simulink model "AEBMIL"  (Simulink 8.2)
settings: Solver=FixedStepDiscrete  StartTime=0.0  StopTime=126  FixedStep=0.005  RelTol=1e-3
PostLoadFcn:
  | , if any(exist('dsrtsu_mdlpostloadfcn', 'file') == [2, 3, 6]), try dsrtsu_mdlpostloadfcn('Execute', bdroot); catch fprintf('Error in PostLoadFcn (dsrtsu_mdlpostloadfcn) for model "%s":\n %s\n', bdroot, lasterr); end, end,
values from neighbouring files (symbols this model uses):
  C_TASK_5MS_S = (	C_TICK_TIME_S      	)    [hcu_local_hdr.m]
  ENUM_GEARPOSN_1ST = uint8(  1  )    [hcu_local_hdr.m]
  ENUM_GEARPOSN_R = uint8(  7  )    [hcu_local_hdr.m]
  FALSE = boolean( 0 )    [hcu_local_hdr.m]
  R_OBJ_Position = single([ii 0 0])    [GridSearch.m]
  R_OBJ_RelAccel = single([0 0 kk])    [GridSearch.m]
  R_OBJ_RelVelocity = single([0 jj 0])    [GridSearch.m]
  TRUE = boolean( 1 )    [hcu_local_hdr.m]
undefined symbols (not defined in the file or in its folder): A_OBJ, AAEB_VehSpd_kph, B_OBJ, C_OBJ, Gamma_OBJ, KAEB_AEBActiveCount_cnt, KAEB_DsblAEBAPPRateThres_pctps, KAEB_DsblAEBSteerRateThres_degps, KAEB_UseMCTTTC_flg, KAEB_VehHoldSpdThres_kph, KOBJ_KalmanFilterCalRate_s, KOBJ_UseCalObjSpd_flg, KOBJ_UseEstObjInfo_flg, KOBJ_VehAccCalRate_s, KOBJ_VehAccFltConst_s, KPTH_ObjPositionYLimit_m, MAEB_AEBTTCThres_s, MAEB_FCWTTCOffset_s, magnitude, MPTH_TurningRadius_m, Q_OBJ, slcm
libraries: simulink x49, hcu_lib x22, dspmtrx3 x3, dspinverses x1
(part 3 of 3)

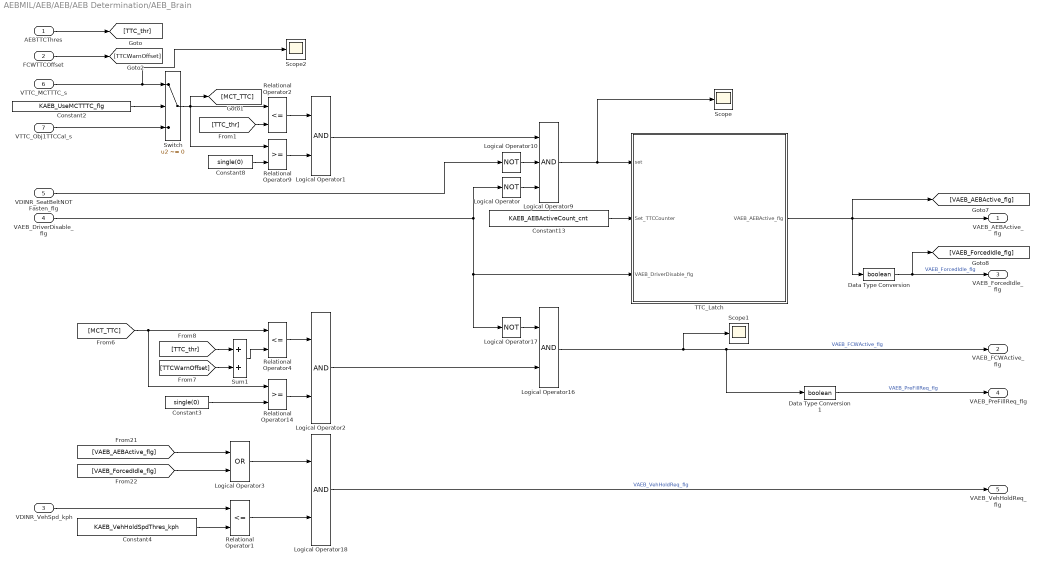
== system AEBMIL/AEB/AEB/AEB Determination/AEB_Brain ==
  AEBTTCThres : Inport
  FCWTTCOffset : Inport  Port=2
  VDINR_VehSpd_kph : Inport  Port=3
  VAEB_DriverDisable_flg : Inport  Port=4
  VDINR_SeatBeltNOTFasten_flg : Inport  Port=5
  VTTC_MCTTTC_s : Inport  Port=6
  VTTC_Obj1TTCCal_s : Inport  Port=7
  Constant13 : Constant  Value=KAEB_AEBActiveCount_cnt
  Constant2 : Constant  Value=KAEB_UseMCTTTC_flg
  Constant3 : Constant  Value=single(0)
  Constant4 : Constant  Value=KAEB_VehHoldSpdThres_kph
  Constant8 : Constant  Value=single(0)
  Data Type Conversion : DataTypeConversion  OutDataTypeStr=boolean
  Data Type Conversion1 : DataTypeConversion  OutDataTypeStr=boolean
  Logical Operator : Logic  Operator=NOT  AllPortsSameDT=off  OutDataTypeStr=boolean
  Logical Operator{1..2,16,18} (4 alike) : Logic  AllPortsSameDT=off  OutDataTypeStr=boolean
  Logical Operator10 : Logic  Operator=NOT  AllPortsSameDT=off  OutDataTypeStr=boolean
  Logical Operator17 : Logic  Operator=NOT  AllPortsSameDT=off  OutDataTypeStr=boolean
  Logical Operator3 : Logic  Operator=OR  AllPortsSameDT=off  OutDataTypeStr=boolean
  Logical Operator9 : Logic  Inputs=3  AllPortsSameDT=off  OutDataTypeStr=boolean
  Relational Operator1 : RelationalOperator  Operator=<=  OutDataTypeStr=boolean
  Relational Operator14 : RelationalOperator  OutDataTypeStr=boolean
  Relational Operator2 : RelationalOperator  Operator=<=  OutDataTypeStr=boolean
  Relational Operator4 : RelationalOperator  Operator=<=  OutDataTypeStr=boolean
  Relational Operator9 : RelationalOperator  OutDataTypeStr=boolean
  Scope : Scope
  Scope1 : Scope
  Scope2 : Scope
      settings: SaveName=ScopeData16
  Sum1 : Sum
  Switch : Switch  Criteria=u2 ~= 0
  TTC_Latch : Subsystem
  VAEB_AEBActive_flg : Outport
  VAEB_FCWActive_flg : Outport  Port=2
  VAEB_ForcedIdle_flg : Outport  Port=3
  VAEB_PreFillReq_flg : Outport  Port=4
  VAEB_VehHoldReq_flg : Outport  Port=5
  wires:
  Logical Operator18/1 -> VAEB_VehHoldReq_flg/1  "VAEB_VehHoldReq_flg"
  Constant4/1 -> Relational Operator1/2
  VDINR_VehSpd_kph/1 -> Relational Operator1/1
  Relational Operator1/1 -> Logical Operator18/2
  Logical Operator3/1 -> Logical Operator18/1
  [VAEB_ForcedIdle_flg] -> Logical Operator3/2
  [VAEB_AEBActive_flg] -> Logical Operator3/1
  Data Type Conversion1/1 -> VAEB_PreFillReq_flg/1  "VAEB_PreFillReq_flg"
  Data Type Conversion/1 -> VAEB_ForcedIdle_flg/1, [VAEB_ForcedIdle_flg]  "VAEB_ForcedIdle_flg"
  Logical Operator16/1 -> Scope1/1, Data Type Conversion1/1, VAEB_FCWActive_flg/1  "VAEB_FCWActive_flg"
  Logical Operator17/1 -> Logical Operator16/1
  Logical Operator2/1 -> Logical Operator16/2
  Constant3/1 -> Relational Operator14/2
  Sum1/1 -> Relational Operator4/2
  [MCT_TTC] -> Relational Operator4/1, Relational Operator14/1
  Relational Operator4/1 -> Logical Operator2/1
  Relational Operator14/1 -> Logical Operator2/2
  [TTCWarnOffset] -> Sum1/2
  [TTC_thr] -> Sum1/1
  FCWTTCOffset/1 -> [TTCWarnOffset]
  TTC_Latch/1(VAEB_AEBActive_flg) -> Data Type Conversion/1, VAEB_AEBActive_flg/1, [VAEB_AEBActive_flg]
  Logical Operator10/1 -> Logical Operator9/2
  VDINR_SeatBeltNOTFasten_flg/1 -> Logical Operator10/1
  Constant13/1 -> TTC_Latch/2(Set_TTCCounter)
  Logical Operator9/1 -> Scope/1, TTC_Latch/1(set)
  Logical Operator/1 -> Logical Operator9/3
  VAEB_DriverDisable_flg/1 -> Logical Operator17/1, TTC_Latch/3(VAEB_DriverDisable_flg), Logical Operator/1
  Logical Operator1/1 -> Logical Operator9/1
  Relational Operator2/1 -> Logical Operator1/1
  Relational Operator9/1 -> Logical Operator1/2
  Constant8/1 -> Relational Operator9/2
  [TTC_thr] -> Relational Operator2/2
  Switch/1 -> Relational Operator2/1, Relational Operator9/1, [MCT_TTC]
  VTTC_Obj1TTCCal_s/1 -> Switch/3
  VTTC_MCTTTC_s/1 -> Scope2/1, Switch/1
  Constant2/1 -> Switch/2
  AEBTTCThres/1 -> [TTC_thr]

== system AEBMIL/AEB/AEB/Driver Disable/APPRateCalculation ==
  VDINR_HWAccelPedalPosn_pct : Inport
  VDINR_HWAccelPedalPosnValid_flg : Inport  Port=2
  trig_STEERINTEND : TriggerPort  TriggerType=function-call
  Constant : Constant  Value=single(1)
  Constant1 : Constant  Value=single(0)
  Product : Product  Inputs=*/  RndMeth=Zero
  Sum : Sum  Inputs=+-
  Switch : Switch  Criteria=u2 ~= 0
  Unit Delay : UnitDelay  SampleTime=-1
  VAEB_APPMovingRate_pctps : Outport
  wires:
  VDINR_HWAccelPedalPosn_pct/1 -> Sum/1, Unit Delay/1
  Constant/1 -> Product/2
  Sum/1 -> Product/1
  Unit Delay/1 -> Sum/2
  VDINR_HWAccelPedalPosnValid_flg/1 -> Switch/2
  Product/1 -> Switch/1
  Switch/1 -> VAEB_APPMovingRate_pctps/1  "VAEB_APPMovingRate_pctps"
  Constant1/1 -> Switch/3

== system AEBMIL/AEB/AEB/Driver Disable/SteeringRateCalculation ==
  VDINR_SteerAngle_deg : Inport
  VDINR_SteerAngleValid_flg : Inport  Port=2
  trig_STEERINTEND : TriggerPort  TriggerType=function-call
  Constant : Constant  Value=single(1)
  Constant1 : Constant  Value=single(0)
  Product : Product  Inputs=*/  RndMeth=Zero
  Sum : Sum  Inputs=+-
  Switch : Switch  Criteria=u2 ~= 0
  Unit Delay : UnitDelay  SampleTime=-1
  VAEB_SteeringRate_degps : Outport
  wires:
  Constant1/1 -> Switch/3
  Switch/1 -> VAEB_SteeringRate_degps/1  "VAEB_SteeringRate_degps"
  Product/1 -> Switch/1
  VDINR_SteerAngleValid_flg/1 -> Switch/2
  Unit Delay/1 -> Sum/2
  Sum/1 -> Product/1
  Constant/1 -> Product/2
  VDINR_SteerAngle_deg/1 -> Unit Delay/1, Sum/1

== system AEBMIL/OBJ/OBJ/KalmanFilter_Obj1/Kalman Filter ==
  A : Inport
  B : Inport  Port=2
  C : Inport  Port=3
  Yk : Inport  Port=4
  u(k-1) : Inport  Port=5
  Gamma : Inport  Port=6
  Q : Inport  Port=7
  R : Inport  Port=8
  x_hat(k-1|k-1) : Inport  Port=9
  P(k-1|k-1) : Inport  Port=10
  Kalman Gain module : Subsystem
  Matrix Multiply{,1..3} (4 alike) : Product  Multiplication=Matrix(*)
  Sum1 : Sum  Inputs=|+-
  Sum2 : Sum  Inputs=|++
  Sum3 : Sum  Inputs=|++
  x_hat(k|k) : Outport
  P(k|k) : Outport  Port=2
  wires:
  A/1 -> Matrix Multiply/1, Kalman Gain module/1(A)
  x_hat(k-1|k-1)/1 -> Matrix Multiply/2
  Matrix Multiply/1 -> Sum2/1
  B/1 -> Matrix Multiply1/1
  u(k-1)/1 -> Matrix Multiply1/2
  Matrix Multiply1/1 -> Sum2/2
  Yk/1 -> Sum1/1
  C/1 -> Matrix Multiply2/1, Kalman Gain module/2(C)
  Sum2/1 -> Matrix Multiply2/2, Sum3/2  "x_hat(k|k-1)"
  Matrix Multiply2/1 -> Sum1/2
  Kalman Gain module/2(Kalman Gain) -> Matrix Multiply3/1
  Sum1/1 -> Matrix Multiply3/2
  Matrix Multiply3/1 -> Sum3/1
  Sum3/1 -> x_hat(k|k)/1
  Gamma/1 -> Kalman Gain module/3(Gamma)
  Q/1 -> Kalman Gain module/4(Q)
  R/1 -> Kalman Gain module/5(R)
  Kalman Gain module/1(P(k|k)) -> P(k|k)/1
  P(k-1|k-1)/1 -> Kalman Gain module/6(P(k-1|k-1))

== system AEBMIL/OBJ/OBJ/Obj1_RelVelocity_Calculation/DataPass_Obj1 ==
  In1 : Inport
  Enable : EnablePort  StatesWhenEnabling=reset
  Out1 : Outport  OutputWhenDisabled=reset  InitialOutput=[0]
  wires:
  In1/1 -> Out1/1

== system AEBMIL/OBJ/OBJ/Obj1_RelVelocity_Calculation/Obj1_RelVelocity_Cal ==
  ObjPositionX_m : Inport
  TimeDur_s : Inport  Port=2
  Trigger : TriggerPort
  Compare To Zero1 : simulink/Logic and Bit Operations/Compare To Zero  relop=~=  OutDataTypeStr=boolean
  Compare To Zero2 : simulink/Logic and Bit Operations/Compare To Zero  relop=~=  OutDataTypeStr=boolean
  Compare To Zero3 : simulink/Logic and Bit Operations/Compare To Zero  relop=~=  OutDataTypeStr=boolean
  Constant1 : Constant  Value=0  OutDataTypeStr=single
  Enabled Subsystem : Subsystem  TreatAsAtomicUnit=on
  Logical Operator : Logic  Inputs=3  AllPortsSameDT=off  OutDataTypeStr=boolean
  Sum : Sum  Inputs=+-
  Unit Delay : UnitDelay  SampleTime=-1
  Unit Delay2 : UnitDelay  SampleTime=-1
  divide : hcu_lib/divide
  VOBJ_Obj1RelVelocityCal_mps : Outport
  wires:
  Unit Delay2/1 -> Compare To Zero3/1
  Compare To Zero3/1 -> Logical Operator/3
  Enabled Subsystem/1(Out1) -> divide/1
  Sum/1 -> Enabled Subsystem/1(In1)
  Logical Operator/1 -> Enabled Subsystem/Enable
  Compare To Zero2/1 -> Logical Operator/2
  Compare To Zero1/1 -> Logical Operator/1
  Constant1/1 -> divide/3
  TimeDur_s/1 -> divide/2
  ObjPositionX_m/1 -> Unit Delay/1, Sum/1, Compare To Zero1/1
  Unit Delay/1 -> Sum/2, Unit Delay2/1, Compare To Zero2/1
  divide/1 -> VOBJ_Obj1RelVelocityCal_mps/1  "VOBJ_Obj1RelVelocityCal_mps"

== system AEBMIL/OBJ/OBJ/Obj1_RelVelocity_Calculation/SandH_Obj1 ==
  In1 : Inport
  Trigger : TriggerPort
  Out1 : Outport
  wires:
  In1/1 -> Out1/1

== system AEBMIL/OBJ/OBJ/Obj1_RelVelocity_Calculation/Timer1 ==
  Enable : EnablePort  StatesWhenEnabling=reset  ZeroCross=off
  Constant : Constant  Value=C_TASK_5MS_S
  Sum : Sum  Inputs=|++  SaturateOnIntegerOverflow=on  InputSameDT=on
  Unit Delay : UnitDelay  SampleTime=-1
  Timer (sec) : Outport  OutputWhenDisabled=reset  InitialOutput=0
  wires:
  Constant/1 -> Sum/1
  Sum/1 -> Unit Delay/1
  Unit Delay/1 -> Sum/2, Timer (sec)/1

== system AEBMIL/OBJ/OBJ/Obj2_RelVelocity_Calculation/DataPass_Obj2 ==
  In1 : Inport
  Enable : EnablePort  StatesWhenEnabling=reset
  Out1 : Outport  OutputWhenDisabled=reset  InitialOutput=[0]
  wires:
  In1/1 -> Out1/1

== system AEBMIL/OBJ/OBJ/Obj2_RelVelocity_Calculation/Obj2_RelVelocity_Cal ==
  ObjPositionX_m : Inport
  TimeDur_s : Inport  Port=2
  Trigger : TriggerPort
  Compare To Zero1 : simulink/Logic and Bit Operations/Compare To Zero  relop=~=  OutDataTypeStr=boolean
  Compare To Zero2 : simulink/Logic and Bit Operations/Compare To Zero  relop=~=  OutDataTypeStr=boolean
  Compare To Zero3 : simulink/Logic and Bit Operations/Compare To Zero  relop=~=  OutDataTypeStr=boolean
  Constant1 : Constant  Value=0  OutDataTypeStr=single
  Enabled Subsystem : Subsystem  TreatAsAtomicUnit=on
  Logical Operator : Logic  Inputs=3  AllPortsSameDT=off  OutDataTypeStr=boolean
  Sum : Sum  Inputs=+-
  Unit Delay : UnitDelay  SampleTime=-1
  Unit Delay2 : UnitDelay  SampleTime=-1
  divide : hcu_lib/divide
  VOBJ_Obj2RelVelocityCal_mps : Outport
  wires:
  divide/1 -> VOBJ_Obj2RelVelocityCal_mps/1  "VOBJ_Obj2RelVelocityCal_mps"
  Unit Delay/1 -> Compare To Zero2/1, Unit Delay2/1, Sum/2
  ObjPositionX_m/1 -> Compare To Zero1/1, Sum/1, Unit Delay/1
  TimeDur_s/1 -> divide/2
  Constant1/1 -> divide/3
  Compare To Zero1/1 -> Logical Operator/1
  Compare To Zero2/1 -> Logical Operator/2
  Logical Operator/1 -> Enabled Subsystem/Enable
  Sum/1 -> Enabled Subsystem/1(In1)
  Enabled Subsystem/1(Out1) -> divide/1
  Compare To Zero3/1 -> Logical Operator/3
  Unit Delay2/1 -> Compare To Zero3/1

== system AEBMIL/OBJ/OBJ/Obj2_RelVelocity_Calculation/SandH_Obj2 ==
  In1 : Inport
  Trigger : TriggerPort
  Out1 : Outport
  wires:
  In1/1 -> Out1/1

== system AEBMIL/OBJ/OBJ/Obj2_RelVelocity_Calculation/Timer2 ==
  Enable : EnablePort  StatesWhenEnabling=reset  ZeroCross=off
  Constant : Constant  Value=C_TASK_5MS_S
  Sum : Sum  Inputs=|++  SaturateOnIntegerOverflow=on  InputSameDT=on
  Unit Delay : UnitDelay  SampleTime=-1
  Timer (sec) : Outport  OutputWhenDisabled=reset  InitialOutput=0
  wires:
  Unit Delay/1 -> Timer (sec)/1, Sum/2
  Sum/1 -> Unit Delay/1
  Constant/1 -> Sum/1

== system AEBMIL/OBJ/OBJ/Obj3_RelVelocity_Calculation/DataPass_Obj3 ==
  In1 : Inport
  Enable : EnablePort  StatesWhenEnabling=reset
  Out1 : Outport  OutputWhenDisabled=reset  InitialOutput=[0]
  wires:
  In1/1 -> Out1/1

== system AEBMIL/OBJ/OBJ/Obj3_RelVelocity_Calculation/Obj3_RelVelocity_Cal ==
  ObjPositionX_m : Inport
  TimeDur_s : Inport  Port=2
  Trigger : TriggerPort
  Compare To Zero1 : simulink/Logic and Bit Operations/Compare To Zero  relop=~=  OutDataTypeStr=boolean
  Compare To Zero2 : simulink/Logic and Bit Operations/Compare To Zero  relop=~=  OutDataTypeStr=boolean
  Compare To Zero3 : simulink/Logic and Bit Operations/Compare To Zero  relop=~=  OutDataTypeStr=boolean
  Constant1 : Constant  Value=0  OutDataTypeStr=single
  Enabled Subsystem : Subsystem  TreatAsAtomicUnit=on
  Logical Operator : Logic  Inputs=3  AllPortsSameDT=off  OutDataTypeStr=boolean
  Sum : Sum  Inputs=+-
  Unit Delay : UnitDelay  SampleTime=-1
  Unit Delay2 : UnitDelay  SampleTime=-1
  divide : hcu_lib/divide
  VOBJ_Obj3RelVelocityCal_mps : Outport
  wires:
  Unit Delay2/1 -> Compare To Zero3/1
  Compare To Zero3/1 -> Logical Operator/3
  Enabled Subsystem/1(Out1) -> divide/1
  Sum/1 -> Enabled Subsystem/1(In1)
  Logical Operator/1 -> Enabled Subsystem/Enable
  Compare To Zero2/1 -> Logical Operator/2
  Compare To Zero1/1 -> Logical Operator/1
  Constant1/1 -> divide/3
  TimeDur_s/1 -> divide/2
  ObjPositionX_m/1 -> Unit Delay/1, Sum/1, Compare To Zero1/1
  Unit Delay/1 -> Sum/2, Unit Delay2/1, Compare To Zero2/1
  divide/1 -> VOBJ_Obj3RelVelocityCal_mps/1  "VOBJ_Obj3RelVelocityCal_mps"

== system AEBMIL/OBJ/OBJ/Obj3_RelVelocity_Calculation/SandH_Obj3 ==
  In1 : Inport
  Trigger : TriggerPort
  Out1 : Outport
  wires:
  In1/1 -> Out1/1

== system AEBMIL/OBJ/OBJ/Obj3_RelVelocity_Calculation/Timer3 ==
  Enable : EnablePort  StatesWhenEnabling=reset  ZeroCross=off
  Constant : Constant  Value=C_TASK_5MS_S
  Sum : Sum  Inputs=|++  SaturateOnIntegerOverflow=on  InputSameDT=on
  Unit Delay : UnitDelay  SampleTime=-1
  Timer (sec) : Outport  OutputWhenDisabled=reset  InitialOutput=0
  wires:
  Constant/1 -> Sum/1
  Sum/1 -> Unit Delay/1
  Unit Delay/1 -> Sum/2, Timer (sec)/1

== system AEBMIL/OBJ/OBJ/Obj4_RelVelocity_Calculation/DataPass_Obj4 ==
  In1 : Inport
  Enable : EnablePort  StatesWhenEnabling=reset
  Out1 : Outport  OutputWhenDisabled=reset  InitialOutput=[0]
  wires:
  In1/1 -> Out1/1

== system AEBMIL/OBJ/OBJ/Obj4_RelVelocity_Calculation/Obj4_RelVelocity_Cal ==
  ObjPositionX_m : Inport
  TimeDur_s : Inport  Port=2
  Trigger : TriggerPort
  Compare To Zero1 : simulink/Logic and Bit Operations/Compare To Zero  relop=~=  OutDataTypeStr=boolean
  Compare To Zero2 : simulink/Logic and Bit Operations/Compare To Zero  relop=~=  OutDataTypeStr=boolean
  Compare To Zero3 : simulink/Logic and Bit Operations/Compare To Zero  relop=~=  OutDataTypeStr=boolean
  Constant1 : Constant  Value=0  OutDataTypeStr=single
  Enabled Subsystem : Subsystem  TreatAsAtomicUnit=on
  Logical Operator : Logic  Inputs=3  AllPortsSameDT=off  OutDataTypeStr=boolean
  Sum : Sum  Inputs=+-
  Unit Delay : UnitDelay  SampleTime=-1
  Unit Delay2 : UnitDelay  SampleTime=-1
  divide : hcu_lib/divide
  VOBJ_Obj4RelVelocityCal_mps : Outport
  wires:
  divide/1 -> VOBJ_Obj4RelVelocityCal_mps/1  "VOBJ_Obj4RelVelocityCal_mps"
  Unit Delay/1 -> Compare To Zero2/1, Unit Delay2/1, Sum/2
  ObjPositionX_m/1 -> Compare To Zero1/1, Sum/1, Unit Delay/1
  TimeDur_s/1 -> divide/2
  Constant1/1 -> divide/3
  Compare To Zero1/1 -> Logical Operator/1
  Compare To Zero2/1 -> Logical Operator/2
  Logical Operator/1 -> Enabled Subsystem/Enable
  Sum/1 -> Enabled Subsystem/1(In1)
  Enabled Subsystem/1(Out1) -> divide/1
  Compare To Zero3/1 -> Logical Operator/3
  Unit Delay2/1 -> Compare To Zero3/1

== system AEBMIL/OBJ/OBJ/Obj4_RelVelocity_Calculation/SandH_Obj4 ==
  In1 : Inport
  Trigger : TriggerPort
  Out1 : Outport
  wires:
  In1/1 -> Out1/1

== system AEBMIL/OBJ/OBJ/Obj4_RelVelocity_Calculation/Timer4 ==
  Enable : EnablePort  StatesWhenEnabling=reset  ZeroCross=off
  Constant : Constant  Value=C_TASK_5MS_S
  Sum : Sum  Inputs=|++  SaturateOnIntegerOverflow=on  InputSameDT=on
  Unit Delay : UnitDelay  SampleTime=-1
  Timer (sec) : Outport  OutputWhenDisabled=reset  InitialOutput=0
  wires:
  Unit Delay/1 -> Timer (sec)/1, Sum/2
  Sum/1 -> Unit Delay/1
  Constant/1 -> Sum/1

== system AEBMIL/OBJ/OBJ/Obj5_RelVelocity_Calculation/DataPass_Obj5 ==
  In1 : Inport
  Enable : EnablePort  StatesWhenEnabling=reset
  Out1 : Outport  OutputWhenDisabled=reset  InitialOutput=[0]
  wires:
  In1/1 -> Out1/1

== system AEBMIL/OBJ/OBJ/Obj5_RelVelocity_Calculation/Obj5_RelVelocity_Cal ==
  ObjPositionX_m : Inport
  TimeDur_s : Inport  Port=2
  Trigger : TriggerPort
  Compare To Zero1 : simulink/Logic and Bit Operations/Compare To Zero  relop=~=  OutDataTypeStr=boolean
  Compare To Zero2 : simulink/Logic and Bit Operations/Compare To Zero  relop=~=  OutDataTypeStr=boolean
  Compare To Zero3 : simulink/Logic and Bit Operations/Compare To Zero  relop=~=  OutDataTypeStr=boolean
  Constant1 : Constant  Value=0  OutDataTypeStr=single
  Enabled Subsystem : Subsystem  TreatAsAtomicUnit=on
  Logical Operator : Logic  Inputs=3  AllPortsSameDT=off  OutDataTypeStr=boolean
  Sum : Sum  Inputs=+-
  Unit Delay : UnitDelay  SampleTime=-1
  Unit Delay2 : UnitDelay  SampleTime=-1
  divide : hcu_lib/divide
  VOBJ_Obj5RelVelocityCal_mps : Outport
  wires:
  Unit Delay2/1 -> Compare To Zero3/1
  Compare To Zero3/1 -> Logical Operator/3
  Enabled Subsystem/1(Out1) -> divide/1
  Sum/1 -> Enabled Subsystem/1(In1)
  Logical Operator/1 -> Enabled Subsystem/Enable
  Compare To Zero2/1 -> Logical Operator/2
  Compare To Zero1/1 -> Logical Operator/1
  Constant1/1 -> divide/3
  TimeDur_s/1 -> divide/2
  ObjPositionX_m/1 -> Unit Delay/1, Sum/1, Compare To Zero1/1
  Unit Delay/1 -> Sum/2, Unit Delay2/1, Compare To Zero2/1
  divide/1 -> VOBJ_Obj5RelVelocityCal_mps/1  "VOBJ_Obj5RelVelocityCal_mps"

== system AEBMIL/OBJ/OBJ/Obj5_RelVelocity_Calculation/SandH_Obj5 ==
  In1 : Inport
  Trigger : TriggerPort
  Out1 : Outport
  wires:
  In1/1 -> Out1/1

== system AEBMIL/OBJ/OBJ/Obj5_RelVelocity_Calculation/Timer5 ==
  Enable : EnablePort  StatesWhenEnabling=reset  ZeroCross=off
  Constant : Constant  Value=C_TASK_5MS_S
  Sum : Sum  Inputs=|++  SaturateOnIntegerOverflow=on  InputSameDT=on
  Unit Delay : UnitDelay  SampleTime=-1
  Timer (sec) : Outport  OutputWhenDisabled=reset  InitialOutput=0
  wires:
  Constant/1 -> Sum/1
  Sum/1 -> Unit Delay/1
  Unit Delay/1 -> Sum/2, Timer (sec)/1

== system AEBMIL/OBJ/OBJ/Trigger signal generator/trigger signal generator ==
  Time_dur [s] : Inport
  Constant3 : Constant  Value=0  OutDataTypeStr=single
  Constant4 : Constant  Value=C_TASK_5MS_S
  Relational Operator1 : RelationalOperator  OutDataTypeStr=boolean
  Sum1 : Sum  Inputs=|++  SaturateOnIntegerOverflow=on  InputSameDT=on
  Sum2 : Sum  Inputs=+-
  Switch3 : Switch  Threshold=0.5
  Unit Delay2 : UnitDelay  SampleTime=-1
  Unit Delay3 : UnitDelay  SampleTime=-1
  Trigger_signal : Outport  OutputWhenDisabled=reset  InitialOutput=[0]
  wires:
  Sum2/1 -> Relational Operator1/2
  Unit Delay3/1 -> Switch3/2
  Unit Delay2/1 -> Sum1/2
  Switch3/1 -> Relational Operator1/1, Unit Delay2/1
  Constant3/1 -> Switch3/1
  Time_dur [s]/1 -> Sum2/1
  Relational Operator1/1 -> Unit Delay3/1, Trigger_signal/1
  Constant4/1 -> Sum2/2, Sum1/1
  Sum1/1 -> Switch3/3

== system AEBMIL/OBJ/OBJ/Trigger signal generator1/trigger signal generator ==
  Time_dur [s] : Inport
  Constant3 : Constant  Value=0  OutDataTypeStr=single
  Constant4 : Constant  Value=C_TASK_5MS_S
  Relational Operator1 : RelationalOperator  OutDataTypeStr=boolean
  Sum1 : Sum  Inputs=|++  SaturateOnIntegerOverflow=on  InputSameDT=on
  Sum2 : Sum  Inputs=+-
  Switch3 : Switch  Threshold=0.5
  Unit Delay2 : UnitDelay  SampleTime=-1
  Unit Delay3 : UnitDelay  SampleTime=-1
  Trigger_signal : Outport  OutputWhenDisabled=reset  InitialOutput=[0]
  wires:
  Sum2/1 -> Relational Operator1/2
  Unit Delay3/1 -> Switch3/2
  Unit Delay2/1 -> Sum1/2
  Switch3/1 -> Relational Operator1/1, Unit Delay2/1
  Constant3/1 -> Switch3/1
  Time_dur [s]/1 -> Sum2/1
  Relational Operator1/1 -> Unit Delay3/1, Trigger_signal/1
  Constant4/1 -> Sum2/2, Sum1/1
  Sum1/1 -> Switch3/3

== system AEBMIL/OBJ/OBJ/Vehicle Acceleration Calculation/signal_filter ==
  raw_input : Inport
  Tc : Inport  Port=2
  Ts : Inport  Port=3
  FirstOrderFilter : Subsystem  RTWFileName=HCU_LIB
      settings: RTWFileNameOpts=User specified
  IC : UnitDelay  Tag=struct('comment',struct('text','','placement',1),'logdata',struct('maxnumvals',inf,'plotchannels',[],'stepsize',0,'downsampling',1,'loggingmode',3,'channels',1),'output',struct('width',1,'name','$S_$B','unit','','type','Int16','offset',0,'max',NaN,'min',NaN,'freeze',1,'lsb',1,'arb',0,'class','default','address','','description','','autoscalingmode',1,'lowerheadroom',1,'upperheadroom',1,'headroomunit','bit','checkmin',0,'checkmax',0,'show',0,'initial','2'),'state',0,'dt','-1','date',731455.586925799)  SampleTime=-1
  Switch1 : Switch  Tag=struct('comment',struct('text','','placement',1),'logdata',struct('maxnumvals',inf,'plotchannels',[],'stepsize',0,'downsampling',1,'loggingmode',3,'channels',1),'output',struct('width',1,'name','$S_$B','unit','','type','Int32Bin15','offset',0,'max',65535,'min',-65536,'freeze',1,'lsb',2^-15,'arb',0,'class','default','address','','description','','autoscalingmode',1,'lowerheadroom',1,'upperheadroom',1,'headroomunit','bit','checkmin',0,'checkmax',0,'show',0),'threshold',struct('width',1,'name','$S_$B_threshold','unit','','type','Int16','offset',0,'max',NaN,'min',NaN,'freeze',1,'lsb',1,'arb',0,'class','default','address','','description','','value','1','scalar',0),'date',731455.58657044)  Threshold=0.5  InputSameDT=on
  zero : Constant  Tag=struct('comment',struct('text','','placement',1),'output',struct('width',1,'name','$S_$B','unit','','type','Int16','offset',0,'max',NaN,'min',NaN,'freeze',1,'lsb',1,'arb',0,'class','default','address','','description','','value','0','tolerance',1,'show',0),'date',731455.58675544)  Value=TRUE
  zero1 : Constant  Tag=struct('comment',struct('text','','placement',1),'output',struct('width',1,'name','$S_$B','unit','','type','Int16','offset',0,'max',NaN,'min',NaN,'freeze',1,'lsb',1,'arb',0,'class','default','address','','description','','value','0','tolerance',1,'show',0),'date',731455.58675544)  Value=0  OutDataTypeStr=single
  raw_input_filt : Outport
  wires:
  zero/1 -> IC/1
  raw_input/1 -> FirstOrderFilter/1(in)
  Tc/1 -> Switch1/1
  Ts/1 -> FirstOrderFilter/3(Ts)
  IC/1 -> Switch1/2
  FirstOrderFilter/1(out) -> raw_input_filt/1
  Switch1/1 -> FirstOrderFilter/2(Tc)
  zero1/1 -> Switch1/3

== system AEBMIL/PTH/PathEstimation/Object in Path/Object1 ==
  VPTH_HostPathYOfstWRTObj1_m : Inport
  VPTH_Obj1WithinRadius_flg : Inport  Port=2
  VTRCK_Obj1PositionY_m : Inport  Port=3
  KPTH_ObjPositionYLimit_m : Inport  Port=4
  Logical Operator : Logic  AllPortsSameDT=off  OutDataTypeStr=boolean
  Logical Operator1 : Logic  AllPortsSameDT=off  OutDataTypeStr=boolean
  Relational Operator : RelationalOperator  Operator=<=  OutDataTypeStr=boolean
  Relational Operator1 : RelationalOperator  Operator=<=  OutDataTypeStr=boolean
  Sum : Sum
  Sum1 : Sum  Inputs=+-
  VPTH_Obj1InPath_flg : Outport
  wires:
  Logical Operator1/1 -> VPTH_Obj1InPath_flg/1  "VPTH_Obj1InPath_flg"
  Logical Operator/1 -> Logical Operator1/1
  VPTH_Obj1WithinRadius_flg/1 -> Logical Operator1/2
  VPTH_HostPathYOfstWRTObj1_m/1 -> Sum1/1, Sum/2
  KPTH_ObjPositionYLimit_m/1 -> Sum1/2, Sum/1
  VTRCK_Obj1PositionY_m/1 -> Relational Operator/2, Relational Operator1/1
  Sum1/1 -> Relational Operator/1
  Sum/1 -> Relational Operator1/2
  Relational Operator1/1 -> Logical Operator/2
  Relational Operator/1 -> Logical Operator/1

== system AEBMIL/PTH/PathEstimation/Object in Path/Object2 ==
  VPTH_HostPathYOfstWRTObj2_m : Inport
  VPTH_Obj2WithinRadius_flg : Inport  Port=2
  VTRCK_Obj2PositionY_m : Inport  Port=3
  KPTH_ObjPositionYLimit_m : Inport  Port=4
  Logical Operator : Logic  AllPortsSameDT=off  OutDataTypeStr=boolean
  Logical Operator1 : Logic  AllPortsSameDT=off  OutDataTypeStr=boolean
  Relational Operator : RelationalOperator  Operator=<=  OutDataTypeStr=boolean
  Relational Operator1 : RelationalOperator  Operator=<=  OutDataTypeStr=boolean
  Sum : Sum
  Sum1 : Sum  Inputs=+-
  VPTH_Obj2InPath_flg : Outport
  wires:
  Relational Operator/1 -> Logical Operator/1
  Relational Operator1/1 -> Logical Operator/2
  Sum/1 -> Relational Operator1/2
  Sum1/1 -> Relational Operator/1
  VTRCK_Obj2PositionY_m/1 -> Relational Operator1/1, Relational Operator/2
  KPTH_ObjPositionYLimit_m/1 -> Sum/1, Sum1/2
  VPTH_HostPathYOfstWRTObj2_m/1 -> Sum/2, Sum1/1
  VPTH_Obj2WithinRadius_flg/1 -> Logical Operator1/2
  Logical Operator/1 -> Logical Operator1/1
  Logical Operator1/1 -> VPTH_Obj2InPath_flg/1  "VPTH_Obj2InPath_flg"

== system AEBMIL/PTH/PathEstimation/Object in Path/Object3 ==
  VPTH_HostPathYOfstWRTObj3_m : Inport
  VPTH_Obj3WithinRadius_flg : Inport  Port=2
  VTRCK_Obj3PositionY_m : Inport  Port=3
  KPTH_ObjPositionYLimit_m : Inport  Port=4
  Logical Operator : Logic  AllPortsSameDT=off  OutDataTypeStr=boolean
  Logical Operator1 : Logic  AllPortsSameDT=off  OutDataTypeStr=boolean
  Relational Operator : RelationalOperator  Operator=<=  OutDataTypeStr=boolean
  Relational Operator1 : RelationalOperator  Operator=<=  OutDataTypeStr=boolean
  Sum : Sum
  Sum1 : Sum  Inputs=+-
  VPTH_Obj3InPath_flg : Outport
  wires:
  Logical Operator1/1 -> VPTH_Obj3InPath_flg/1  "VPTH_Obj3InPath_flg"
  Logical Operator/1 -> Logical Operator1/1
  VPTH_Obj3WithinRadius_flg/1 -> Logical Operator1/2
  VPTH_HostPathYOfstWRTObj3_m/1 -> Sum1/1, Sum/2
  KPTH_ObjPositionYLimit_m/1 -> Sum1/2, Sum/1
  VTRCK_Obj3PositionY_m/1 -> Relational Operator/2, Relational Operator1/1
  Sum1/1 -> Relational Operator/1
  Sum/1 -> Relational Operator1/2
  Relational Operator1/1 -> Logical Operator/2
  Relational Operator/1 -> Logical Operator/1

== system AEBMIL/PTH/PathEstimation/Object in Path/Object4 ==
  VPTH_HostPathYOfstWRTObj4_m : Inport
  VPTH_Obj4WithinRadius_flg : Inport  Port=2
  VTRCK_Obj4PositionY_m : Inport  Port=3
  KPTH_ObjPositionYLimit_m : Inport  Port=4
  Logical Operator : Logic  AllPortsSameDT=off  OutDataTypeStr=boolean
  Logical Operator1 : Logic  AllPortsSameDT=off  OutDataTypeStr=boolean
  Relational Operator : RelationalOperator  Operator=<=  OutDataTypeStr=boolean
  Relational Operator1 : RelationalOperator  Operator=<=  OutDataTypeStr=boolean
  Sum : Sum
  Sum1 : Sum  Inputs=+-
  VPTH_Obj4InPath_flg : Outport
  wires:
  Relational Operator/1 -> Logical Operator/1
  Relational Operator1/1 -> Logical Operator/2
  Sum/1 -> Relational Operator1/2
  Sum1/1 -> Relational Operator/1
  VTRCK_Obj4PositionY_m/1 -> Relational Operator1/1, Relational Operator/2
  KPTH_ObjPositionYLimit_m/1 -> Sum/1, Sum1/2
  VPTH_HostPathYOfstWRTObj4_m/1 -> Sum/2, Sum1/1
  VPTH_Obj4WithinRadius_flg/1 -> Logical Operator1/2
  Logical Operator/1 -> Logical Operator1/1
  Logical Operator1/1 -> VPTH_Obj4InPath_flg/1  "VPTH_Obj4InPath_flg"

== system AEBMIL/PTH/PathEstimation/Object in Path/Object5 ==
  VPTH_HostPathYOfstWRTObj5_m : Inport
  VPTH_Obj5WithinRadius_flg : Inport  Port=2
  VTRCK_Obj5PositionY_m : Inport  Port=3
  KPTH_ObjPositionYLimit_m : Inport  Port=4
  Logical Operator : Logic  AllPortsSameDT=off  OutDataTypeStr=boolean
  Logical Operator1 : Logic  AllPortsSameDT=off  OutDataTypeStr=boolean
  Relational Operator : RelationalOperator  Operator=<=  OutDataTypeStr=boolean
  Relational Operator1 : RelationalOperator  Operator=<=  OutDataTypeStr=boolean
  Sum : Sum
  Sum1 : Sum  Inputs=+-
  VPTH_Obj5InPath_flg : Outport
  wires:
  Logical Operator1/1 -> VPTH_Obj5InPath_flg/1  "VPTH_Obj5InPath_flg"
  Logical Operator/1 -> Logical Operator1/1
  VPTH_Obj5WithinRadius_flg/1 -> Logical Operator1/2
  VPTH_HostPathYOfstWRTObj5_m/1 -> Sum1/1, Sum/2
  KPTH_ObjPositionYLimit_m/1 -> Sum1/2, Sum/1
  VTRCK_Obj5PositionY_m/1 -> Relational Operator/2, Relational Operator1/1
  Sum1/1 -> Relational Operator/1
  Sum/1 -> Relational Operator1/2
  Relational Operator1/1 -> Logical Operator/2
  Relational Operator/1 -> Logical Operator/1

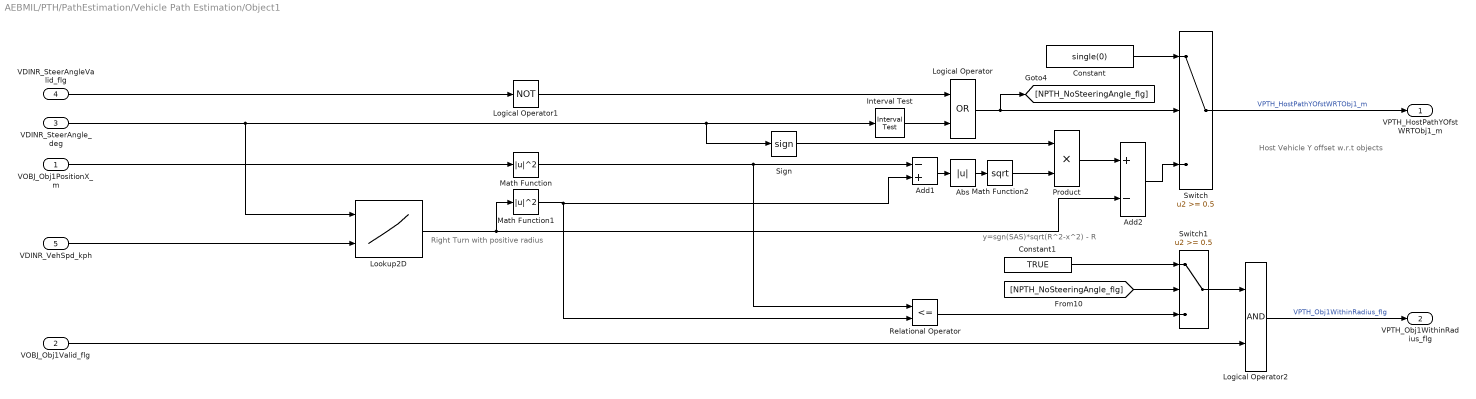
== system AEBMIL/PTH/PathEstimation/Vehicle Path Estimation/Object1 ==
  note: y=sgn(SAS)*sqrt(R^2-x^2) - R
  note: Host Vehicle Y offset w.r.t objects
  note: Right Turn with positive radius
  VOBJ_Obj1PositionX_m : Inport
  VOBJ_Obj1Valid_flg : Inport  Port=2
  VDINR_SteerAngle_deg : Inport  Port=3
  VDINR_SteerAngleValid_flg : Inport  Port=4
  VDINR_VehSpd_kph : Inport  Port=5
  Abs : Abs
  Add1 : Sum  Inputs=-+
  Add2 : Sum  Inputs=+-
  Constant : Constant  Value=single(0)
  Constant1 : Constant  Value=TRUE
  Interval Test : simulink/Logic and Bit Operations/Interval Test  IntervalClosedRight=on  uplimit=10  IntervalClosedLeft=on  lowlimit=-10  OutDataTypeStr=boolean
  Logical Operator : Logic  Operator=OR  AllPortsSameDT=off  OutDataTypeStr=boolean
  Logical Operator1 : Logic  Operator=NOT  AllPortsSameDT=off  OutDataTypeStr=boolean
  Logical Operator2 : Logic  AllPortsSameDT=off  OutDataTypeStr=boolean
  Lookup2D : Lookup2D  RowIndex=APTH_SteerAngle_deg  ColumnIndex=APTH_VehSpd_kph  Table=MPTH_TurningRadius_m  LookUpMeth=Interpolation-Use End Values  OutDataTypeStr=single
      settings: AttributesFormatString=|
      | <row=%<RowIndex>>
      | <column=%<ColumnIndex>>
      | <table=%<Table>>
  Math Function : Math  Operator=magnitude^2  SaturateOnIntegerOverflow=on
  Math Function1 : Math  Operator=magnitude^2  SaturateOnIntegerOverflow=on
  Math Function2 : Math  Operator=sqrt  SaturateOnIntegerOverflow=on
  Product : Product  RndMeth=Zero
  Relational Operator : RelationalOperator  Operator=<=  OutDataTypeStr=boolean
  Sign : Signum
  Switch : Switch  Threshold=0.5
  Switch1 : Switch  Threshold=0.5
  VPTH_HostPathYOfstWRTObj1_m : Outport
  VPTH_Obj1WithinRadius_flg : Outport  Port=2
  wires:
  VOBJ_Obj1Valid_flg/1 -> Logical Operator2/2
  Switch1/1 -> Logical Operator2/1
  Logical Operator1/1 -> Logical Operator/1
  VDINR_SteerAngleValid_flg/1 -> Logical Operator1/1
  Interval Test/1 -> Logical Operator/2
  VDINR_SteerAngle_deg/1 -> Sign/1, Interval Test/1, Lookup2D/1
  Lookup2D/1 -> Math Function1/1, Add2/2
  Sign/1 -> Product/1
  Product/1 -> Add2/1
  VDINR_VehSpd_kph/1 -> Lookup2D/2
  VOBJ_Obj1PositionX_m/1 -> Math Function/1
  Logical Operator/1 -> Switch/2, [NPTH_NoSteeringAngle_flg]
  Switch/1 -> VPTH_HostPathYOfstWRTObj1_m/1  "VPTH_HostPathYOfstWRTObj1_m"
  Add2/1 -> Switch/3
  Constant/1 -> Switch/1
  Math Function/1 -> Add1/1, Relational Operator/1
  Math Function1/1 -> Add1/2, Relational Operator/2
  Add1/1 -> Abs/1
  Math Function2/1 -> Product/2
  Relational Operator/1 -> Switch1/3
  Logical Operator2/1 -> VPTH_Obj1WithinRadius_flg/1  "VPTH_Obj1WithinRadius_flg"
  Constant1/1 -> Switch1/1
  Abs/1 -> Math Function2/1
  [NPTH_NoSteeringAngle_flg] -> Switch1/2

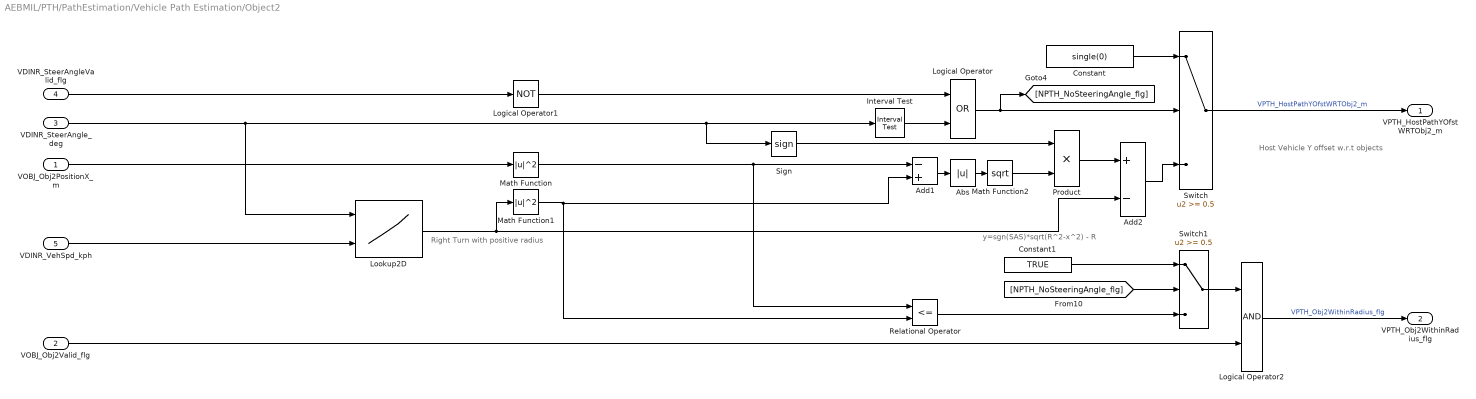
== system AEBMIL/PTH/PathEstimation/Vehicle Path Estimation/Object2 ==
  note: Right Turn with positive radius
  note: Host Vehicle Y offset w.r.t objects
  note: y=sgn(SAS)*sqrt(R^2-x^2) - R
  VOBJ_Obj2PositionX_m : Inport
  VOBJ_Obj2Valid_flg : Inport  Port=2
  VDINR_SteerAngle_deg : Inport  Port=3
  VDINR_SteerAngleValid_flg : Inport  Port=4
  VDINR_VehSpd_kph : Inport  Port=5
  Abs : Abs
  Add1 : Sum  Inputs=-+
  Add2 : Sum  Inputs=+-
  Constant : Constant  Value=single(0)
  Constant1 : Constant  Value=TRUE
  Interval Test : simulink/Logic and Bit Operations/Interval Test  IntervalClosedRight=on  uplimit=10  IntervalClosedLeft=on  lowlimit=-10  OutDataTypeStr=boolean
  Logical Operator : Logic  Operator=OR  AllPortsSameDT=off  OutDataTypeStr=boolean
  Logical Operator1 : Logic  Operator=NOT  AllPortsSameDT=off  OutDataTypeStr=boolean
  Logical Operator2 : Logic  AllPortsSameDT=off  OutDataTypeStr=boolean
  Lookup2D : Lookup2D  RowIndex=APTH_SteerAngle_deg  ColumnIndex=APTH_VehSpd_kph  Table=MPTH_TurningRadius_m  LookUpMeth=Interpolation-Use End Values  OutDataTypeStr=single
      settings: AttributesFormatString=|
      | <row=%<RowIndex>>
      | <column=%<ColumnIndex>>
      | <table=%<Table>>
  Math Function : Math  Operator=magnitude^2  SaturateOnIntegerOverflow=on
  Math Function1 : Math  Operator=magnitude^2  SaturateOnIntegerOverflow=on
  Math Function2 : Math  Operator=sqrt  SaturateOnIntegerOverflow=on
  Product : Product  RndMeth=Zero
  Relational Operator : RelationalOperator  Operator=<=  OutDataTypeStr=boolean
  Sign : Signum
  Switch : Switch  Threshold=0.5
  Switch1 : Switch  Threshold=0.5
  VPTH_HostPathYOfstWRTObj2_m : Outport
  VPTH_Obj2WithinRadius_flg : Outport  Port=2
  wires:
  VOBJ_Obj2Valid_flg/1 -> Logical Operator2/2
  Switch1/1 -> Logical Operator2/1
  Logical Operator1/1 -> Logical Operator/1
  [NPTH_NoSteeringAngle_flg] -> Switch1/2
  Abs/1 -> Math Function2/1
  Constant1/1 -> Switch1/1
  Logical Operator2/1 -> VPTH_Obj2WithinRadius_flg/1  "VPTH_Obj2WithinRadius_flg"
  Relational Operator/1 -> Switch1/3
  Math Function2/1 -> Product/2
  Add1/1 -> Abs/1
  Math Function1/1 -> Relational Operator/2, Add1/2
  Math Function/1 -> Relational Operator/1, Add1/1
  Constant/1 -> Switch/1
  Add2/1 -> Switch/3
  Switch/1 -> VPTH_HostPathYOfstWRTObj2_m/1  "VPTH_HostPathYOfstWRTObj2_m"
  Logical Operator/1 -> [NPTH_NoSteeringAngle_flg], Switch/2
  VOBJ_Obj2PositionX_m/1 -> Math Function/1
  VDINR_VehSpd_kph/1 -> Lookup2D/2
  Product/1 -> Add2/1
  Sign/1 -> Product/1
  Lookup2D/1 -> Add2/2, Math Function1/1
  VDINR_SteerAngle_deg/1 -> Lookup2D/1, Interval Test/1, Sign/1
  Interval Test/1 -> Logical Operator/2
  VDINR_SteerAngleValid_flg/1 -> Logical Operator1/1

== system AEBMIL/PTH/PathEstimation/Vehicle Path Estimation/Object3 ==
  note: y=sgn(SAS)*sqrt(R^2-x^2) - R
  note: Host Vehicle Y offset w.r.t objects
  note: Right Turn with positive radius
  VOBJ_Obj3PositionX_m : Inport
  VOBJ_Obj3Valid_flg : Inport  Port=2
  VDINR_SteerAngle_deg : Inport  Port=3
  VDINR_SteerAngleValid_flg : Inport  Port=4
  VDINR_VehSpd_kph : Inport  Port=5
  Abs : Abs
  Add1 : Sum  Inputs=-+
  Add2 : Sum  Inputs=+-
  Constant : Constant  Value=single(0)
  Constant1 : Constant  Value=TRUE
  Interval Test : simulink/Logic and Bit Operations/Interval Test  IntervalClosedRight=on  uplimit=10  IntervalClosedLeft=on  lowlimit=-10  OutDataTypeStr=boolean
  Logical Operator : Logic  Operator=OR  AllPortsSameDT=off  OutDataTypeStr=boolean
  Logical Operator1 : Logic  Operator=NOT  AllPortsSameDT=off  OutDataTypeStr=boolean
  Logical Operator2 : Logic  AllPortsSameDT=off  OutDataTypeStr=boolean
  Lookup2D : Lookup2D  RowIndex=APTH_SteerAngle_deg  ColumnIndex=APTH_VehSpd_kph  Table=MPTH_TurningRadius_m  LookUpMeth=Interpolation-Use End Values  OutDataTypeStr=single
      settings: AttributesFormatString=|
      | <row=%<RowIndex>>
      | <column=%<ColumnIndex>>
      | <table=%<Table>>
  Math Function : Math  Operator=magnitude^2  SaturateOnIntegerOverflow=on
  Math Function1 : Math  Operator=magnitude^2  SaturateOnIntegerOverflow=on
  Math Function2 : Math  Operator=sqrt  SaturateOnIntegerOverflow=on
  Product : Product  RndMeth=Zero
  Relational Operator : RelationalOperator  Operator=<=  OutDataTypeStr=boolean
  Sign : Signum
  Switch : Switch  Threshold=0.5
  Switch1 : Switch  Threshold=0.5
  VPTH_HostPathYOfstWRTObj3_m : Outport
  VPTH_Obj3WithinRadius_flg : Outport  Port=2
  wires:
  VOBJ_Obj3Valid_flg/1 -> Logical Operator2/2
  Switch1/1 -> Logical Operator2/1
  Logical Operator1/1 -> Logical Operator/1
  VDINR_SteerAngleValid_flg/1 -> Logical Operator1/1
  Interval Test/1 -> Logical Operator/2
  VDINR_SteerAngle_deg/1 -> Sign/1, Interval Test/1, Lookup2D/1
  Lookup2D/1 -> Math Function1/1, Add2/2
  Sign/1 -> Product/1
  Product/1 -> Add2/1
  VDINR_VehSpd_kph/1 -> Lookup2D/2
  VOBJ_Obj3PositionX_m/1 -> Math Function/1
  Logical Operator/1 -> Switch/2, [NPTH_NoSteeringAngle_flg]
  Switch/1 -> VPTH_HostPathYOfstWRTObj3_m/1  "VPTH_HostPathYOfstWRTObj3_m"
  Add2/1 -> Switch/3
  Constant/1 -> Switch/1
  Math Function/1 -> Add1/1, Relational Operator/1
  Math Function1/1 -> Add1/2, Relational Operator/2
  Add1/1 -> Abs/1
  Math Function2/1 -> Product/2
  Relational Operator/1 -> Switch1/3
  Logical Operator2/1 -> VPTH_Obj3WithinRadius_flg/1  "VPTH_Obj3WithinRadius_flg"
  Constant1/1 -> Switch1/1
  Abs/1 -> Math Function2/1
  [NPTH_NoSteeringAngle_flg] -> Switch1/2

== system AEBMIL/PTH/PathEstimation/Vehicle Path Estimation/Object4 ==
  note: Right Turn with positive radius
  note: Host Vehicle Y offset w.r.t objects
  note: y=sgn(SAS)*sqrt(R^2-x^2) - R
  VOBJ_Obj4PositionX_m : Inport
  VOBJ_Obj4Valid_flg : Inport  Port=2
  VDINR_SteerAngle_deg : Inport  Port=3
  VDINR_SteerAngleValid_flg : Inport  Port=4
  VDINR_VehSpd_kph : Inport  Port=5
  Abs : Abs
  Add1 : Sum  Inputs=-+
  Add2 : Sum  Inputs=+-
  Constant : Constant  Value=single(0)
  Constant1 : Constant  Value=TRUE
  Interval Test : simulink/Logic and Bit Operations/Interval Test  IntervalClosedRight=on  uplimit=10  IntervalClosedLeft=on  lowlimit=-10  OutDataTypeStr=boolean
  Logical Operator : Logic  Operator=OR  AllPortsSameDT=off  OutDataTypeStr=boolean
  Logical Operator1 : Logic  Operator=NOT  AllPortsSameDT=off  OutDataTypeStr=boolean
  Logical Operator2 : Logic  AllPortsSameDT=off  OutDataTypeStr=boolean
  Lookup2D : Lookup2D  RowIndex=APTH_SteerAngle_deg  ColumnIndex=APTH_VehSpd_kph  Table=MPTH_TurningRadius_m  LookUpMeth=Interpolation-Use End Values  OutDataTypeStr=single
      settings: AttributesFormatString=|
      | <row=%<RowIndex>>
      | <column=%<ColumnIndex>>
      | <table=%<Table>>
  Math Function : Math  Operator=magnitude^2  SaturateOnIntegerOverflow=on
  Math Function1 : Math  Operator=magnitude^2  SaturateOnIntegerOverflow=on
  Math Function2 : Math  Operator=sqrt  SaturateOnIntegerOverflow=on
  Product : Product  RndMeth=Zero
  Relational Operator : RelationalOperator  Operator=<=  OutDataTypeStr=boolean
  Sign : Signum
  Switch : Switch  Threshold=0.5
  Switch1 : Switch  Threshold=0.5
  VPTH_HostPathYOfstWRTObj4_m : Outport
  VPTH_Obj4WithinRadius_flg : Outport  Port=2
  wires:
  VOBJ_Obj4Valid_flg/1 -> Logical Operator2/2
  Switch1/1 -> Logical Operator2/1
  Logical Operator1/1 -> Logical Operator/1
  [NPTH_NoSteeringAngle_flg] -> Switch1/2
  Abs/1 -> Math Function2/1
  Constant1/1 -> Switch1/1
  Logical Operator2/1 -> VPTH_Obj4WithinRadius_flg/1  "VPTH_Obj4WithinRadius_flg"
  Relational Operator/1 -> Switch1/3
  Math Function2/1 -> Product/2
  Add1/1 -> Abs/1
  Math Function1/1 -> Relational Operator/2, Add1/2
  Math Function/1 -> Relational Operator/1, Add1/1
  Constant/1 -> Switch/1
  Add2/1 -> Switch/3
  Switch/1 -> VPTH_HostPathYOfstWRTObj4_m/1  "VPTH_HostPathYOfstWRTObj4_m"
  Logical Operator/1 -> [NPTH_NoSteeringAngle_flg], Switch/2
  VOBJ_Obj4PositionX_m/1 -> Math Function/1
  VDINR_VehSpd_kph/1 -> Lookup2D/2
  Product/1 -> Add2/1
  Sign/1 -> Product/1
  Lookup2D/1 -> Add2/2, Math Function1/1
  VDINR_SteerAngle_deg/1 -> Lookup2D/1, Interval Test/1, Sign/1
  Interval Test/1 -> Logical Operator/2
  VDINR_SteerAngleValid_flg/1 -> Logical Operator1/1

== system AEBMIL/PTH/PathEstimation/Vehicle Path Estimation/Object5 ==
  note: y=sgn(SAS)*sqrt(R^2-x^2) - R
  note: Host Vehicle Y offset w.r.t objects
  note: Right Turn with positive radius
  VOBJ_Obj5PositionX_m : Inport
  VOBJ_Obj5Valid_flg : Inport  Port=2
  VDINR_SteerAngle_deg : Inport  Port=3
  VDINR_SteerAngleValid_flg : Inport  Port=4
  VDINR_VehSpd_kph : Inport  Port=5
  Abs : Abs
  Add1 : Sum  Inputs=-+
  Add2 : Sum  Inputs=+-
  Constant : Constant  Value=single(0)
  Constant1 : Constant  Value=TRUE
  Interval Test : simulink/Logic and Bit Operations/Interval Test  IntervalClosedRight=on  uplimit=10  IntervalClosedLeft=on  lowlimit=-10  OutDataTypeStr=boolean
  Logical Operator : Logic  Operator=OR  AllPortsSameDT=off  OutDataTypeStr=boolean
  Logical Operator1 : Logic  Operator=NOT  AllPortsSameDT=off  OutDataTypeStr=boolean
  Logical Operator2 : Logic  AllPortsSameDT=off  OutDataTypeStr=boolean
  Lookup2D : Lookup2D  RowIndex=APTH_SteerAngle_deg  ColumnIndex=APTH_VehSpd_kph  Table=MPTH_TurningRadius_m  LookUpMeth=Interpolation-Use End Values  OutDataTypeStr=single
      settings: AttributesFormatString=|
      | <row=%<RowIndex>>
      | <column=%<ColumnIndex>>
      | <table=%<Table>>
  Math Function : Math  Operator=magnitude^2  SaturateOnIntegerOverflow=on
  Math Function1 : Math  Operator=magnitude^2  SaturateOnIntegerOverflow=on
  Math Function2 : Math  Operator=sqrt  SaturateOnIntegerOverflow=on
  Product : Product  RndMeth=Zero
  Relational Operator : RelationalOperator  Operator=<=  OutDataTypeStr=boolean
  Sign : Signum
  Switch : Switch  Threshold=0.5
  Switch1 : Switch  Threshold=0.5
  VPTH_HostPathYOfstWRTObj5_m : Outport
  VPTH_Obj5WithinRadius_flg : Outport  Port=2
  wires:
  VOBJ_Obj5Valid_flg/1 -> Logical Operator2/2
  Switch1/1 -> Logical Operator2/1
  Logical Operator1/1 -> Logical Operator/1
  VDINR_SteerAngleValid_flg/1 -> Logical Operator1/1
  Interval Test/1 -> Logical Operator/2
  VDINR_SteerAngle_deg/1 -> Sign/1, Interval Test/1, Lookup2D/1
  Lookup2D/1 -> Math Function1/1, Add2/2
  Sign/1 -> Product/1
  Product/1 -> Add2/1
  VDINR_VehSpd_kph/1 -> Lookup2D/2
  VOBJ_Obj5PositionX_m/1 -> Math Function/1
  Logical Operator/1 -> Switch/2, [NPTH_NoSteeringAngle_flg]
  Switch/1 -> VPTH_HostPathYOfstWRTObj5_m/1  "VPTH_HostPathYOfstWRTObj5_m"
  Add2/1 -> Switch/3
  Constant/1 -> Switch/1
  Math Function/1 -> Add1/1, Relational Operator/1
  Math Function1/1 -> Add1/2, Relational Operator/2
  Add1/1 -> Abs/1
  Math Function2/1 -> Product/2
  Relational Operator/1 -> Switch1/3
  Logical Operator2/1 -> VPTH_Obj5WithinRadius_flg/1  "VPTH_Obj5WithinRadius_flg"
  Constant1/1 -> Switch1/1
  Abs/1 -> Math Function2/1
  [NPTH_NoSteeringAngle_flg] -> Switch1/2

== system AEBMIL/AEB/AEB/AEB Determination/AEB_Brain/TTC_Latch ==
  set : Inport
  Set_TTCCounter : Inport  Port=2
  VAEB_DriverDisable_flg : Inport  Port=3
  Counter : Subsystem
  Relational Opertor2 : RelationalOperator  Operator=>  OutDataTypeStr=boolean
  SR_Latch : Subsystem
  VAEB_AEBActive_flg : Outport
  wires:
  VAEB_DriverDisable_flg/1 -> SR_Latch/2(reset), Counter/2(reset)
  SR_Latch/1(latched) -> VAEB_AEBActive_flg/1  "VAEB_AEBActive_flg"
  Relational Opertor2/1 -> SR_Latch/1(set)
  Set_TTCCounter/1 -> Relational Opertor2/2
  Counter/1(count) -> Relational Opertor2/1
  set/1 -> Counter/1(trigger)

== system AEBMIL/OBJ/OBJ/KalmanFilter_Obj1/Kalman Filter/Kalman Gain module ==
  A : Inport
  C : Inport  Port=2
  Gamma : Inport  Port=3
  Q : Inport  Port=4
  R : Inport  Port=5
  P(k-1|k-1) : Inport  Port=6
  " LU Inverse" : dspinverses/ LU Inverse
  Matrix Multiply{,1..4} (5 alike) : Product  Inputs=3  Multiplication=Matrix(*)
  Sum : Sum  Inputs=|++
  Sum1 : Sum  Inputs=|+-
  Sum2 : Sum  Inputs=|++
  Transpose : dspmtrx3/Transpose  Hermitian=off  overflowFlag=on
  Transpose1 : dspmtrx3/Transpose  Hermitian=off  overflowFlag=on
  Transpose2 : dspmtrx3/Transpose  Hermitian=off  overflowFlag=on
  P(k|k) : Outport
  Kalman Gain : Outport  Port=2
  wires:
  C/1 -> Transpose/1, Matrix Multiply1/1, Matrix Multiply2/2
  Transpose/1 -> Matrix Multiply/2, Matrix Multiply1/3
  Matrix Multiply1/1 -> Sum/1
  R/1 -> Sum/2
  Sum/1 -> " LU Inverse"/1
  " LU Inverse"/1 -> Matrix Multiply/3
  Matrix Multiply/1 -> Matrix Multiply2/1, Kalman Gain/1
  Matrix Multiply2/1 -> Sum1/2
  A/1 -> Transpose1/1, Matrix Multiply3/1
  Transpose1/1 -> Matrix Multiply3/3
  Matrix Multiply3/1 -> Sum2/1
  Transpose2/1 -> Matrix Multiply4/3
  Gamma/1 -> Transpose2/1, Matrix Multiply4/1
  Q/1 -> Matrix Multiply4/2
  Matrix Multiply4/1 -> Sum2/2
  Sum2/1 -> Matrix Multiply/1, Matrix Multiply1/2, Sum1/1, Matrix Multiply2/3  "P(k|k-1)"
  P(k-1|k-1)/1 -> Matrix Multiply3/2
  Sum1/1 -> P(k|k)/1  "P(k|k)"

== system AEBMIL/OBJ/OBJ/Obj1_RelVelocity_Calculation/Obj1_RelVelocity_Cal/Enabled Subsystem ==
  In1 : Inport
  Enable : EnablePort  StatesWhenEnabling=reset
  Out1 : Outport  OutputWhenDisabled=reset  InitialOutput=[0]
  wires:
  In1/1 -> Out1/1

== system AEBMIL/OBJ/OBJ/Obj2_RelVelocity_Calculation/Obj2_RelVelocity_Cal/Enabled Subsystem ==
  In1 : Inport
  Enable : EnablePort  StatesWhenEnabling=reset
  Out1 : Outport  OutputWhenDisabled=reset  InitialOutput=[0]
  wires:
  In1/1 -> Out1/1

== system AEBMIL/OBJ/OBJ/Obj3_RelVelocity_Calculation/Obj3_RelVelocity_Cal/Enabled Subsystem ==
  In1 : Inport
  Enable : EnablePort  StatesWhenEnabling=reset
  Out1 : Outport  OutputWhenDisabled=reset  InitialOutput=[0]
  wires:
  In1/1 -> Out1/1

== system AEBMIL/OBJ/OBJ/Obj4_RelVelocity_Calculation/Obj4_RelVelocity_Cal/Enabled Subsystem ==
  In1 : Inport
  Enable : EnablePort  StatesWhenEnabling=reset
  Out1 : Outport  OutputWhenDisabled=reset  InitialOutput=[0]
  wires:
  In1/1 -> Out1/1

== system AEBMIL/OBJ/OBJ/Obj5_RelVelocity_Calculation/Obj5_RelVelocity_Cal/Enabled Subsystem ==
  In1 : Inport
  Enable : EnablePort  StatesWhenEnabling=reset
  Out1 : Outport  OutputWhenDisabled=reset  InitialOutput=[0]
  wires:
  In1/1 -> Out1/1

== system AEBMIL/OBJ/OBJ/Vehicle Acceleration Calculation/signal_filter/FirstOrderFilter ==
  in : Inport
  Tc : Inport  Port=2
  Ts : Inport  Port=3
  Add : Sum
  Add1 : Sum
  Add2 : Sum  Inputs=+-
  Constant : Constant  OutDataTypeStr=single
  Divide : Product  Inputs=*/
  Product : Product  RndMeth=Zero
  Product1 : Product  RndMeth=Zero
  Unit Delay : UnitDelay  SampleTime=-1
  out : Outport
  wires:
  Add/1 -> Unit Delay/1, out/1
  Product1/1 -> Add/2
  Product/1 -> Add/1
  Add2/1 -> Product/2
  in/1 -> Product/1
  Divide/1 -> Product1/1, Add2/2
  Constant/1 -> Add2/1
  Add1/1 -> Divide/2
  Ts/1 -> Add1/2
  Tc/1 -> Divide/1, Add1/1
  Unit Delay/1 -> Product1/2

== system AEBMIL/AEB/AEB/AEB Determination/AEB_Brain/TTC_Latch/Counter ==
  trigger : Inport
  reset : Inport  Port=2
  Constant6 : Constant  OutDataTypeStr=single
  Constant7 : Constant  Value=0  OutDataTypeStr=single
  Logical Operator : Logic  AllPortsSameDT=off  OutDataTypeStr=boolean
  Logical Operator1 : Logic  Operator=NOT  AllPortsSameDT=off  OutDataTypeStr=boolean
  Subtract1 : Sum
  Switch1 : Switch  Criteria=u2 ~= 0
  Switch2 : Switch  Criteria=u2 ~= 0
  Unit Delay : UnitDelay  SampleTime=-1
  Unit Delay2 : UnitDelay  SampleTime=-1
  count : Outport
  wires:
  Logical Operator1/1 -> Logical Operator/2
  Logical Operator/1 -> Switch1/2
  reset/1 -> Switch2/2, Logical Operator1/1
  trigger/1 -> Logical Operator/1
  Unit Delay/1 -> Subtract1/1
  Unit Delay2/1 -> Switch2/3
  Constant7/1 -> Switch2/1
  Switch2/1 -> Switch1/3
  Switch1/1 -> count/1, Unit Delay/1, Unit Delay2/1
  Subtract1/1 -> Switch1/1
  Constant6/1 -> Subtract1/2

== system AEBMIL/AEB/AEB/AEB Determination/AEB_Brain/TTC_Latch/SR_Latch ==
  note: 0
  note: 1
  note: 0
  note: 1
  note: 1
  note: 1
  set : Inport
  reset : Inport  Port=2
  Logical Operator : Logic  AllPortsSameDT=off  OutDataTypeStr=boolean
  Logical Operator1 : Logic  Operator=NOT  AllPortsSameDT=off  OutDataTypeStr=boolean
  Switch1 : Switch  Criteria=u2 ~= 0  Threshold=0.5
      settings: AttributesFormatString=<Criteria=%<Criteria>>
  Switch2 : Switch  Criteria=u2 ~= 0  Threshold=0.5
      settings: AttributesFormatString=<Criteria=%<Criteria>>
  Unit Delay : UnitDelay  SampleTime=-1
  latched : Outport
  wires:
  Switch1/1 -> Unit Delay/1, latched/1
  set/1 -> Switch1/1, Logical Operator/1
  reset/1 -> Switch2/2, Logical Operator1/1
  Unit Delay/1 -> Switch2/3
  Switch2/1 -> Switch1/3
  Logical Operator/1 -> Switch1/2
  Logical Operator1/1 -> Logical Operator/2, Switch2/1

== stateflow chart Scheduler ==
  (default) -> (junction 10)
  (junction 10) -> (junction 11) : {
      | trig_DINR; ...
      | trig_TRCK; ...
      | trig_OBJ; ...
      | trig_PTH; ...
      | trig_MCT;...
      | trig_TTC; ...
      | trig_AEB; ...
      | }
  events: trig_DINR output FUNCTION_CALL_EVENT; trig_TRCK output FUNCTION_CALL_EVENT; trig_OBJ output FUNCTION_CALL_EVENT; trig_PTH output FUNCTION_CALL_EVENT; trig_MCT output FUNCTION_CALL_EVENT; trig_TTC output FUNCTION_CALL_EVENT; trig_AEB output FUNCTION_CALL_EVENT

== stateflow chart AEB/AEB/Driver Disable/Function-Call Generator ==
  settings: sampleTime=0.003125
  (default) -> (junction 20)
  (junction 20) -> (junction 21) : {
      | b500ms_count = b500ms_count +1; ...
      | b1000ms_count = b1000ms_count +1; ...
      | }
  (junction 21) -> (junction 22) [order 1] : [b500ms_count == 100]
  (junction 21) -> (junction 23) [order 2]
  (junction 22) -> (junction 24) : /*500ms*/
      | {
      | b500ms_count = 0; ...
      | }
  (junction 24) -> (junction 23)
  (junction 23) -> (junction 25)
  (junction 25) -> (junction 26) [order 1] : [b1000ms_count == 200]
  (junction 25) -> (junction 27) [order 2]
  (junction 26) -> (junction 28) : /*1000ms*/
      | {
      | b1000ms_count = 0; ...
      | trig_STEERINTEND; ...
      | trig_APPINTEND; ...
      | }
  (junction 28) -> (junction 27)
  data: b500ms_count local uint8; b1000ms_count local double
  events: trig_STEERINTEND output FUNCTION_CALL_EVENT; trig_APPINTEND output FUNCTION_CALL_EVENT
